simulink model "m1"  (R2022a)
settings: Solver=VariableStepAuto  StartTime=0.0  StopTime=100*T  RelTol=1e-3
values from neighbouring files (symbols this model uses):
  Kv = 0.03    [autocalibrate.m]    (also in discret_line_system.m = 0.0012)
  m = 0.3    [autocalibrate.m]
  r = 0.2    [autocalibrate.m]
  T = 0.05    [autocalibrate.m]    (also in discret_line_system.m = 0.01; hallspeedsence.m = 5e-05)
undefined symbols (not defined in the file or in its folder): DiscIntNeverNeededParam, g
settings Model: Creator=anyus  LastModifiedBy=anyus

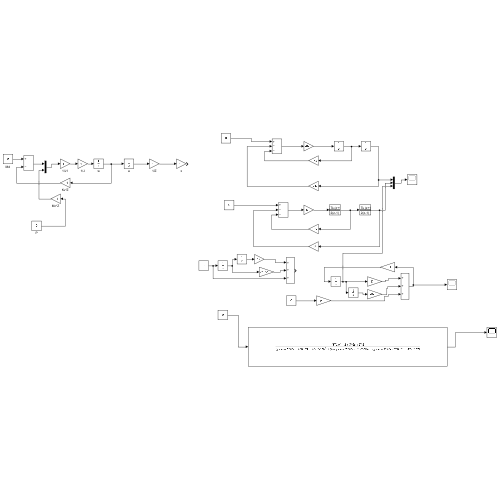
[thumbnail: Simulink's stored preview of the top-level diagram]
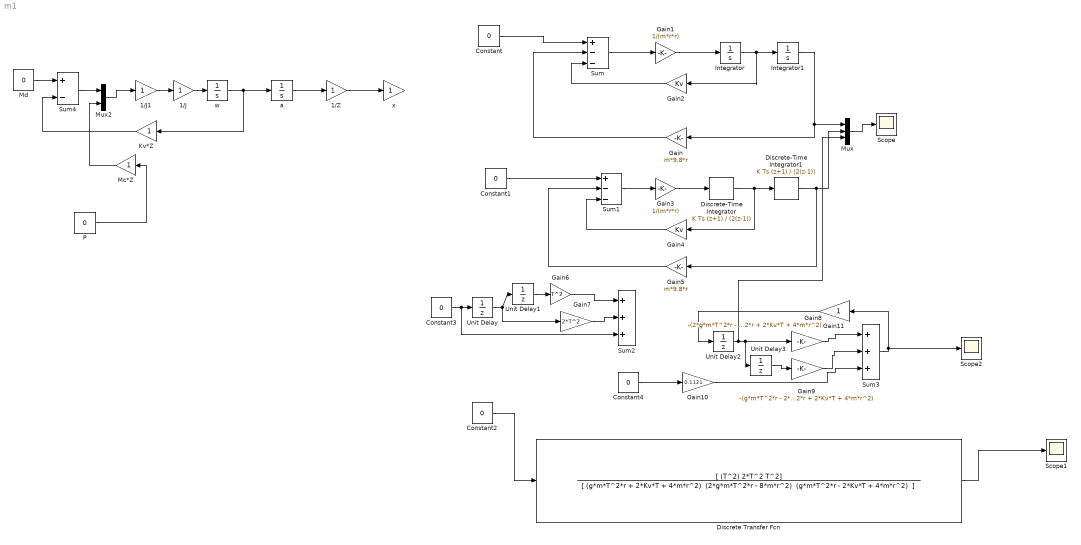
== system m1 ==
  1/J : Gain
  1/J1 : Gain
  1/Z : Gain
  Constant{,1..3} (4 alike) : Constant  Value=0
  Constant4 : Constant  Value=0  SampleTime=T
  Discrete Transfer Fcn : DiscreteTransferFcn  Numerator=[ (T^2) 2*T^2 T^2]  Denominator="[ (g*m*T^2*r + 2*Kv*T + 4*m*r^2)  (2*g*m*T^2*r - 8*m*r^2)  (g*m*T^2*r - 2*Kv*T + 4*m*r^2)  ]"  InitialStates=pi/6  SampleTime=T
  Discrete-Time Integrator : DiscreteIntegrator  IntegratorMethod=Integration: Trapezoidal  SampleTime=T  ICPrevOutput=DiscIntNeverNeededParam  ICPrevScaledInput=DiscIntNeverNeededParam
  Discrete-Time Integrator1 : DiscreteIntegrator  IntegratorMethod=Integration: Trapezoidal  InitialCondition=pi/6  SampleTime=T  ICPrevOutput=DiscIntNeverNeededParam  ICPrevScaledInput=DiscIntNeverNeededParam
  Gain : Gain  Gain=m*9.8*r
  Gain1 : Gain  Gain=1/(m*r*r)
  Gain10 : Gain  Gain=0.1121
  Gain11 : Gain
  Gain2 : Gain  Gain=Kv
  Gain3 : Gain  Gain=1/(m*r*r)
  Gain4 : Gain  Gain=Kv
  Gain5 : Gain  Gain=m*9.8*r
  Gain6 : Gain  Gain=T^2
  Gain7 : Gain  Gain=2*T^2
  Gain8 : Gain  Gain=-(2*g*m*T^2*r - 8*m*r^2)/(g*m*T^2*r + 2*Kv*T + 4*m*r^2)
  Gain9 : Gain  Gain=-(g*m*T^2*r - 2*Kv*T + 4*m*r^2)/(g*m*T^2*r + 2*Kv*T + 4*m*r^2)
  Integrator : Integrator
  Integrator1 : Integrator  InitialCondition=pi/6
  Kv*Z : Gain
  Mc*Z : Gain
  Md : Constant  Value=0
  Mux : Mux  Inputs=3
  Mux2 : Mux  Inputs=2
  P : Constant  Value=0
  Scope : Scope
  Scope1 : Scope
  Scope2 : Scope
  Sum : Sum  Inputs=+--
  Sum1 : Sum  Inputs=+--
  Sum2 : Sum  Inputs=+++
  Sum3 : Sum  Inputs=+++
  Sum4 : Sum  Inputs=+-
  Unit Delay : UnitDelay  SampleTime=T  HasFrameUpgradeWarning=on
  Unit Delay1 : UnitDelay  SampleTime=T  HasFrameUpgradeWarning=on
  Unit Delay2 : UnitDelay  InitialCondition=pi/6  SampleTime=T  HasFrameUpgradeWarning=on
  Unit Delay3 : UnitDelay  InitialCondition=pi/6  SampleTime=T  HasFrameUpgradeWarning=on
  a : Integrator
  w : Integrator
  x : Gain
  wires:
  Integrator/1 -> Gain2/1, Integrator1/1
  Sum/1 -> Gain1/1
  Integrator1/1 -> Mux/1, Gain/1
  Constant/1 -> Sum/1
  Gain1/1 -> Integrator/1
  Gain/1 -> Sum/2
  Gain2/1 -> Sum/3
  Discrete-Time Integrator/1 -> Gain4/1, Discrete-Time Integrator1/1
  Discrete-Time Integrator1/1 -> Mux/2, Gain5/1
  Gain3/1 -> Discrete-Time Integrator/1
  Sum1/1 -> Gain3/1
  Gain4/1 -> Sum1/3
  Constant1/1 -> Sum1/1
  Gain5/1 -> Sum1/2
  Mux/1 -> Scope/1
  Constant2/1 -> Discrete Transfer Fcn/1
  Discrete Transfer Fcn/1 -> Scope1/1
  Constant3/1 -> Sum2/3, Unit Delay/1
  Unit Delay/1 -> Gain7/1, Unit Delay1/1
  Unit Delay1/1 -> Gain6/1
  Gain6/1 -> Sum2/1
  Gain7/1 -> Sum2/2
  Unit Delay2/1 -> Mux/3, Unit Delay3/1, Gain8/1
  Unit Delay3/1 -> Gain9/1
  Gain8/1 -> Sum3/1
  Gain9/1 -> Sum3/2
  Sum3/1 -> Gain11/1, Scope2/1
  Gain11/1 -> Unit Delay2/1
  Constant4/1 -> Gain10/1
  Gain10/1 -> Sum3/3
  Md/1 -> Sum4/1
  1/J/1 -> w/1
  1/J1/1 -> 1/J/1
  Sum4/1 -> Mux2/1
  Mux2/1 -> 1/J1/1
  Mc*Z/1 -> Mux2/2
  P/1 -> Mc*Z/1
  w/1 -> a/1, Kv*Z/1
  Kv*Z/1 -> Sum4/2
  a/1 -> 1/Z/1
  1/Z/1 -> x/1
